simulink model "servo_final"  (R2020b)
settings: Solver=FixedStepDiscrete  StartTime=0.0  StopTime=Inf  FixedStep=0.001  RelTol=1e-3  EnableMultiTasking=on
values from neighbouring files (symbols this model uses):
  Gtd = c2d(Gt,T,'Tustin')    [demo.m]    (also in pendulo_modelo.m)
  Robs = [1 0 ... (first row only)    [demo.m]    (also in pendulo_modelo.m)
undefined symbols (not defined in the file or in its folder): DiscIntNeverNeededParam, Discrete, Kservo2, Time
libraries: simulink x2, arduinolib x2, ctrlSharedLib x1
settings Model: SILPILModeSetting=veronly  ExtModeTrigDuration=2  Creator=aleca  LastModifiedBy=aleca
settings OptimizationCC: EnhancedBackFolding=on  PassReuseOutputArgsAs=Individual arguments  ZeroExternalMemoryAtStartup=off  ZeroInternalMemoryAtStartup=off  MaxStackSize=64  OptimizeBlockOrder=speed  DifferentSizesBufferReuse=on  OptimizationCustomize=off  EfficientTunableParamExpr=on
settings DebuggingCC: ParameterTunabilityLossMsg=error
settings HardwareCC: ProdBitPerInt=16  ProdBitPerPointer=16  ProdBitPerSizeT=16  ProdBitPerPtrDiffT=16  ProdLargestAtomicFloat=None  ProdWordSize=8  ProdHWDeviceType=Atmel->AVR  UseEmbeddedCoderFeatures=off  UseSimulinkCoderFeatures=off
settings SFSimCC: MATLABDynamicMemAlloc=off
settings RTWCC: Description=Embedded Coder  SystemTargetFile=ert.tlc  HardwareBoard=Arduino Mega 2560  TemplateMakefile=ert_default_tmf  Toolchain=Arduino AVR  BuildConfiguration=Faster Runs
settings CodeAppCC: ForceParamTrailComments=on  IgnoreCustomStorageClasses=off  OperatorAnnotations=on  SimulinkDataObjDesc=on  SFDataObjDesc=on  InsertBlockDesc=on
settings ERTTargetCC: SupportContinuousTime=on  SupportNonInlinedSFcns=on  SupportVariableSizeSignals=on  ExtModeStaticAllocSize=2048

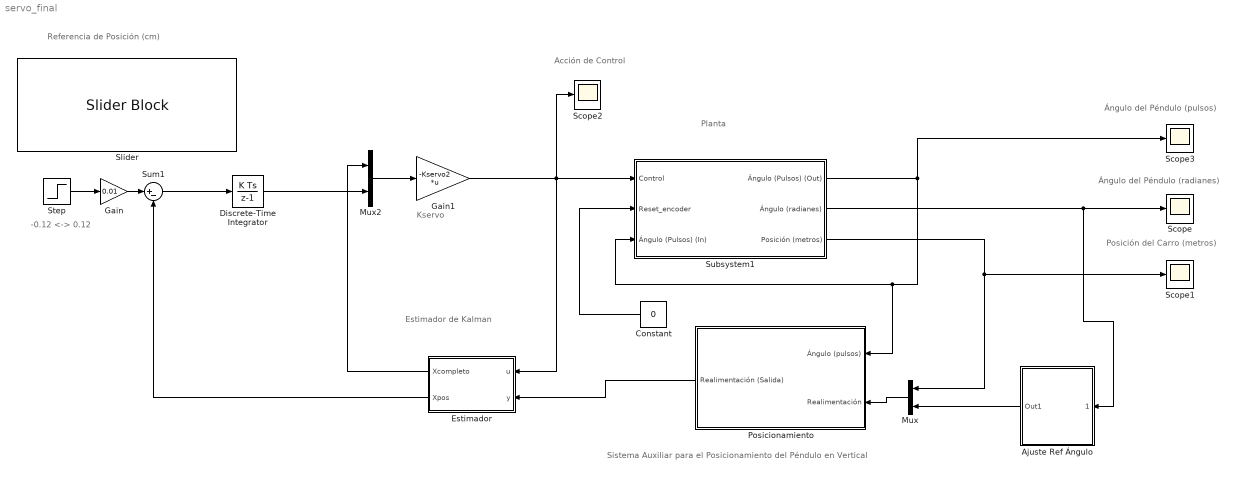
== system servo_final ==
  note: Kservo
  note: Referencia de Posición (cm)
  note: -0.12 <-> 0.12
  note: Planta
  note: Acción de Control
  note: Posición del Carro (metros)
  note: Ángulo del Péndulo (radianes)
  note: Sistema Auxiliar para el Posicionamiento del Péndulo en Vertical
  note: Ángulo del Péndulo (pulsos)
  note: Estimador de
      | Kalman
  Ajuste Ref Ángulo : Subsystem
  Constant : Constant  Value=0  OutDataTypeStr=boolean  SampleTime=0.001
  Discrete-Time Integrator : DiscreteIntegrator  SampleTime=-1  ICPrevOutput=DiscIntNeverNeededParam  ICPrevScaledInput=DiscIntNeverNeededParam
  Estimador : Subsystem
  Gain : Gain  Gain=0.01
  Gain1 : Gain  Gain=-Kservo2  Multiplication=Matrix(K*u)
  Mux : Mux  Inputs=2
  Mux2 : Mux  Inputs=2
  Posicionamiento : Subsystem
  Scope{,1..3} (4 alike) : Scope
  Slider : SliderBlock  ScaleMin=-12  ScaleMax=12  TickInterval=1
  Step : Step  After=0  SampleTime=0.001
  Subsystem1 : Subsystem
  Sum1 : Sum  Inputs=|+-
  wires:
  Subsystem1/1(Ángulo (Pulsos) (Out)) -> Subsystem1/3(Ángulo (Pulsos) (In)), Posicionamiento/1(Ángulo (pulsos)), Scope3/1
  Subsystem1/3(Posición (metros)) -> Scope1/1, Mux/1
  Subsystem1/2(Ángulo (radianes)) -> Ajuste Ref Ángulo/1(1), Scope/1
  Gain1/1 -> Estimador/1(u), Scope2/1, Subsystem1/1(Control)
  Mux/1 -> Posicionamiento/2(Realimentación)
  Sum1/1 -> Discrete-Time Integrator/1
  Step/1 -> Gain/1
  Gain/1 -> Sum1/1
  Discrete-Time Integrator/1 -> Mux2/2
  Mux2/1 -> Gain1/1
  Posicionamiento/1(Realimentación (Salida)) -> Estimador/2(y)
  Estimador/1(Xcompleto) -> Mux2/1
  Estimador/2(Xpos) -> Sum1/2
  Constant/1 -> Subsystem1/2(Reset_encoder)
  Ajuste Ref Ángulo/1(Out1) -> Mux/2

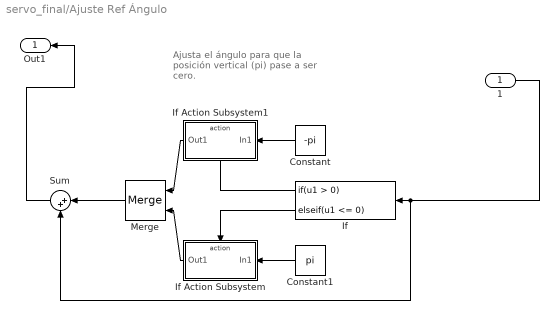
== system servo_final/Ajuste Ref Ángulo ==
  note: Ajusta el ángulo para que la posición vertical (pi) pase a ser cero.
  1 : Inport
  Constant : Constant  Value=-pi  SampleTime=0.001
  Constant1 : Constant  Value=pi  SampleTime=0.001
  If : If  ElseIfExpressions=u1 <= 0  ShowElse=off
  If Action Subsystem : Subsystem  TreatAsAtomicUnit=on
  If Action Subsystem1 : Subsystem  TreatAsAtomicUnit=on
  Merge : Merge
  Sum : Sum  Inputs=|++
  Out1 : Outport
  wires:
  Sum/1 -> Out1/1
  If Action Subsystem/1(Out1) -> Merge/2
  Constant/1 -> If Action Subsystem1/1(In1)
  If Action Subsystem1/1(Out1) -> Merge/1
  If/2 -> If Action Subsystem/Action
  Merge/1 -> Sum/1
  Constant1/1 -> If Action Subsystem/1(In1)
  If/1 -> If Action Subsystem1/Action
  1/1 -> Sum/2, If/1

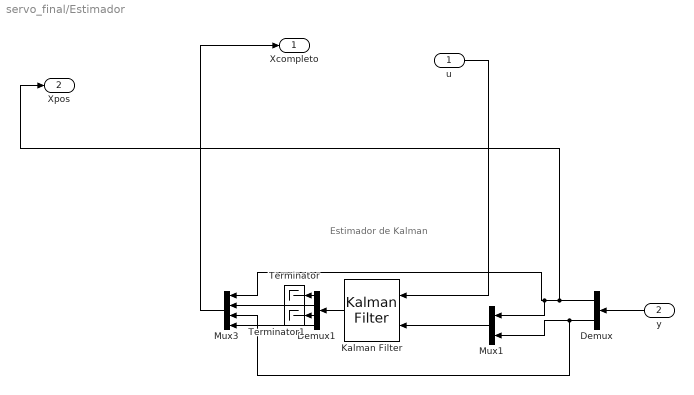
== system servo_final/Estimador ==
  note: Estimador
      | de Kalman
  u : Inport
  y : Inport  Port=2
  Demux : Demux  Outputs=2
  Demux1 : Demux
  Kalman Filter : ctrlSharedLib/Kalman Filter  TimeDomain=Discrete-Time  UseCurrentEstimator=off  ModelSource=Individual A, B, C, D matrices  ModelSourceVariable=ss(0.95,1,1,0,1)  A=Gtd.A  B=Gtd.B  C=Gtd.C  D=Gtd.D  NumberOfStates=1  NumberOfInputs=1  NumberOfOutputs=1  InitialEstimateSource=Dialog  X0=0  P0=10  UseK=off  UseGH=off  NumberOfProcessNoiseInputs=1  G=1  TimeInvariantG=on  H=0  TimeInvariantH=on  Q=Qobs  TimeInvariantQ=on  R=Robs  TimeInvariantR=on  N=0  TimeInvariantN=on  AddInputPort=on  AddEnablePort=off  OutputEstimatedY=off  OutputP=off  Ts=-1
  Mux1 : Mux  Inputs=2
  Mux3 : Mux
  Terminator : Terminator
  Terminator1 : Terminator
  Xcompleto : Outport
  Xpos : Outport  Port=2
  wires:
  Mux3/1 -> Xcompleto/1
  y/1 -> Demux/1
  Demux/1 -> Mux3/1, Mux1/1, Xpos/1
  Demux1/1 -> Terminator/1
  u/1 -> Kalman Filter/1
  Demux1/4 -> Mux3/4
  Kalman Filter/1 -> Demux1/1
  Demux1/2 -> Mux3/2
  Demux1/3 -> Terminator1/1
  Mux1/1 -> Kalman Filter/2
  Demux/2 -> Mux3/3, Mux1/2

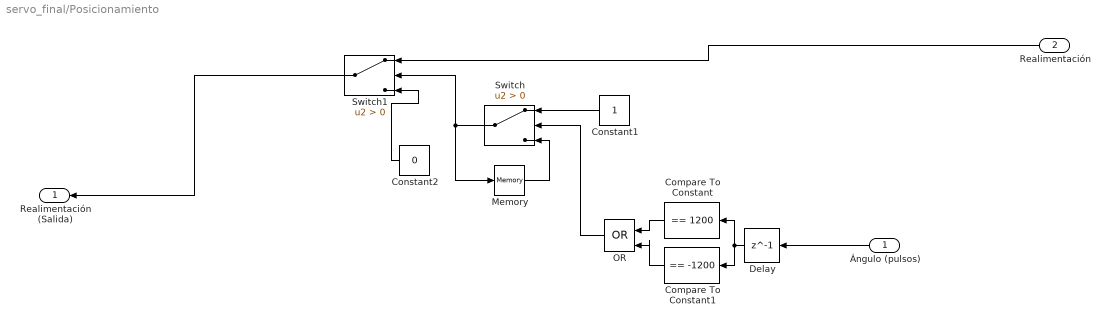
== system servo_final/Posicionamiento ==
  Ángulo (pulsos) : Inport
  Realimentación : Inport  Port=2
  Compare To Constant : simulink/Logic and Bit Operations/Compare To Constant  relop===  const=1200  OutDataTypeStr=boolean
  Compare To Constant1 : simulink/Logic and Bit Operations/Compare To Constant  relop===  const=-1200  OutDataTypeStr=boolean
  Constant1 : Constant  OutDataTypeStr=boolean  SampleTime=-1
  Constant2 : Constant  Value=0  SampleTime=-1
  Delay : Delay  DelayLength=1
  Memory : Memory  InheritSampleTime=on
  OR : Logic  Operator=OR  IconShape=distinctive  AllPortsSameDT=off  OutDataTypeStr=boolean
  Switch : Switch  Criteria=u2 > Threshold
  Switch1 : Switch  Criteria=u2 > Threshold
  Realimentación (Salida) : Outport
  wires:
  Memory/1 -> Switch/3
  Switch/1 -> Switch1/2, Memory/1
  Compare To Constant1/1 -> OR/2
  Compare To Constant/1 -> OR/1
  Delay/1 -> Compare To Constant/1, Compare To Constant1/1
  Constant2/1 -> Switch1/3
  OR/1 -> Switch/2
  Constant1/1 -> Switch/1
  Switch1/1 -> Realimentación (Salida)/1
  Ángulo (pulsos)/1 -> Delay/1
  Realimentación/1 -> Switch1/1

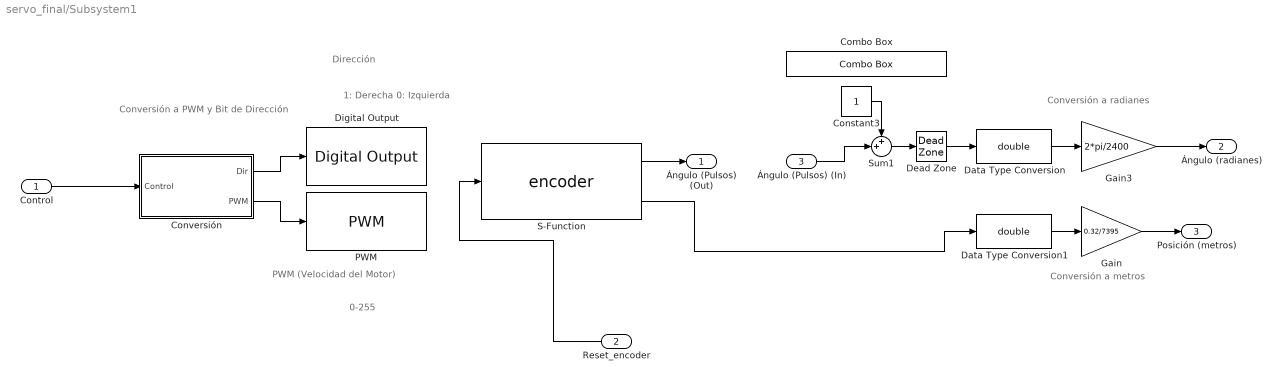
== system servo_final/Subsystem1 ==
  note: Conversión a metros
  note: Dirección
  note: PWM (Velocidad del Motor)
  note: 1: Derecha
      | 0: Izquierda
  note: Conversión a radianes
  note: 0-255
  note: Conversión a PWM y
      | Bit de Dirección
  Control : Inport
  Reset_encoder : Inport  Port=2
  Ángulo (Pulsos) (In) : Inport  Port=3
  Combo Box : ComboBox  LabelPosition=Hide  SelectedLabel=1
      settings: Values={{'0', '1', '2', '-2', '-1'}, [0 1 2 -2 -1]}
  Constant3 : Constant  SampleTime=-1
  Conversión : Subsystem
  Data Type Conversion : DataTypeConversion  OutDataTypeStr=double
  Data Type Conversion1 : DataTypeConversion  OutDataTypeStr=double
  Dead Zone : DeadZone  LowerValue=0  UpperValue=0  SaturateOnIntegerOverflow=on
  Digital Output : arduinolib/Digital Output  pinNumber=10  Direction=output  blockPlatform=arduino
  Gain : Gain  Gain=0.32/7395
  Gain3 : Gain  Gain=2*pi/2400
  PWM : arduinolib/PWM  pinNumber=9  frequencyType=Default  desiredFrequency=490.2  achievableFrequency=490.2
  S-Function : S-Function  FunctionName=encoder  SFunctionModules='encoder_wrapper'  SFunctionDeploymentMode=off  EnableBusSupport=off
  Sum1 : Sum  Inputs=++|
  Ángulo (Pulsos) (Out) : Outport
  Ángulo (radianes) : Outport  Port=2
  Posición (metros) : Outport  Port=3
  wires:
  Gain/1 -> Posición (metros)/1
  Sum1/1 -> Dead Zone/1
  Conversión/1(Dir) -> Digital Output/1
  Conversión/2(PWM) -> PWM/1
  Dead Zone/1 -> Data Type Conversion/1
  Data Type Conversion/1 -> Gain3/1
  Constant3/1 -> Sum1/1
  S-Function/2 -> Data Type Conversion1/1
  Data Type Conversion1/1 -> Gain/1
  S-Function/1 -> Ángulo (Pulsos) (Out)/1
  Reset_encoder/1 -> S-Function/1
  Control/1 -> Conversión/1(Control)
  Gain3/1 -> Ángulo (radianes)/1
  Ángulo (Pulsos) (In)/1 -> Sum1/2

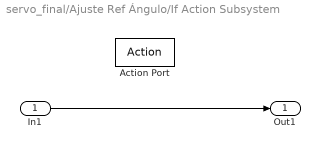
== system servo_final/Ajuste Ref Ángulo/If Action Subsystem ==
  In1 : Inport
  Action Port : ActionPort  ActionPortLabel=elseif(u1 <= 0)
  Out1 : Outport
  wires:
  In1/1 -> Out1/1

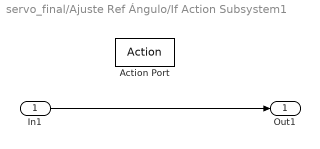
== system servo_final/Ajuste Ref Ángulo/If Action Subsystem1 ==
  In1 : Inport
  Action Port : ActionPort  ActionPortLabel=if(u1 > 0)
  Out1 : Outport
  wires:
  In1/1 -> Out1/1

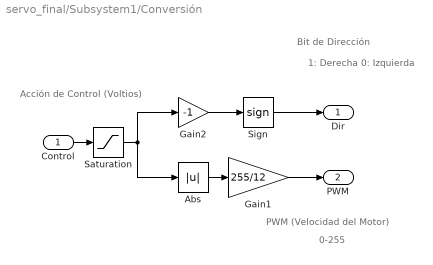
== system servo_final/Subsystem1/Conversión ==
  note: Acción de Control
      | (Voltios)
  note: Bit de Dirección
  note: 1: Derecha
      | 0: Izquierda
  note: 0-255
  note: PWM (Velocidad del Motor)
  Control : Inport
  Abs : Abs
  Gain1 : Gain  Gain=255/12
  Gain2 : Gain  Gain=-1
  Saturation : Saturate  UpperLimit=12  LowerLimit=-12
  Sign : Signum
  Dir : Outport
  PWM : Outport  Port=2
  wires:
  Abs/1 -> Gain1/1
  Gain1/1 -> PWM/1
  Control/1 -> Saturation/1
  Saturation/1 -> Gain2/1, Abs/1
  Sign/1 -> Dir/1
  Gain2/1 -> Sign/1
